simulink library "Fixed_Surface"  (R2018b)
settings: Solver=ode45  StartTime=0.0  StopTime=10.0  RelTol=1e-3  EnableMultiTasking=on
settings Model: Creator=lena.frank  LastModifiedBy=drhf
settings DataIOCC: LimitDataPoints=on  SaveFormat=Array  SignalLoggingSaveFormat=ModelDataLogs
settings OptimizationCC: ExpressionDepthLimit=2147483647  LifeSpan=inf
settings DebuggingCC: UnderspecifiedInitializationDetection=Classic  MergeDetectMultiDrivingBlocksExec=none  SolverPrmCheckMsg=warning  FcnCallInpInsideContextMsg=warning  StateNameClashWarn=warning  SFUnexpectedBacktrackingDiag=warning  SFNoUnconditionalDefaultTransitionDiag=warning  SFExecutionAtInitializationDiag=none
settings HardwareCC: ProdBitPerPointer=32  ProdBitPerSizeT=32  ProdBitPerPtrDiffT=32  ProdLargestAtomicFloat=None  ProdIntDivRoundTo=Undefined  ProdEndianess=Unspecified  ProdWordSize=32  ProdHWDeviceType=32-bit Generic
settings ModelReferenceCC: PropagateSignalLabelsOutOfModel=off
settings SFSimCC: SimUseLocalCustomCode=off
settings RTWCC: RTWUseLocalCustomCode=off
settings CodeAppCC: StateflowObjectComments=on
settings GRTTargetCC: TargetLangStandard=C89/C90 (ANSI)  GeneratePreprocessorConditionals=Disable all  CombineOutputUpdateFcns=off  GRTInterface=on
settings ConfigComp: CovMetricSettings=dw  CovHtmlReporting=on  CovSaveCumulativeToWorkspaceVar=on  CovSaveSingleToWorkspaceVar=on  CovExternalEMLEnable=off

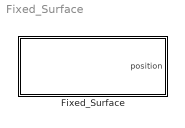
== system Fixed_Surface ==
  Fixed_Surface : Subsystem  mask(fixed surface){colangle=0, colazi=0, colrot=0}
      mask prompts: colangle "Slope of surface (0° = horizontal) [degree]"; colazi "Azimuth of surface (0° = south, -90° = east) [degree]"; colrot "Rotation angle of surface [degree]"
      mask help:
      | Set collector or surface to a fixed position.
      | All angles are limited to the range -180 ° ... +180 °
      mask init:
      | colangle = min(180, max(-180, colangle));
      | colazi = min(180, max(-180, colazi));
      | colrot = min(180, max(-180, colrot));
      mask Help: web(fullfile(path_carnot('help'),'Fixed_Surface.html'),'-helpbrowser')
      mask Display:
      | disp(['Inclination: ' get_param(gcb,'colangle') '°\n\n'])
      | disp(['\n\nAzimuth   : ' get_param(gcb,'colazi') '°\n\n'])
      | disp(['\n\nRotation  : ' get_param(gcb,'colrot') '°'])

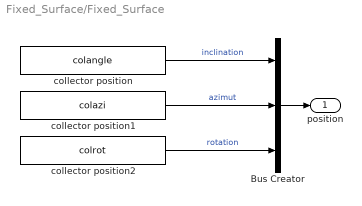
== system Fixed_Surface/Fixed_Surface ==
  Bus Creator : BusCreator  Inputs=3
  collector position : Constant  Value=colangle
  collector position1 : Constant  Value=colazi
  collector position2 : Constant  Value=colrot
  position : Outport
  wires:
  Bus Creator/1 -> position/1
  collector position/1 -> Bus Creator/1  "inclination"
  collector position1/1 -> Bus Creator/2  "azimut"
  collector position2/1 -> Bus Creator/3  "rotation"
